simulink model "siude"  (Simulink 8.5)
settings: Solver=ode4  StartTime=0.0  StopTime=tstop  FixedStep=tstep  RelTol=1e-3
values from neighbouring files (symbols this model uses):
  bs_nom = Ka*Mn*dn*wa    (= -4.53426272631)    [dataude.m]
  kcm = 0.7    [dataude.m]
  kcn = 1.3    [dataude.m]
  rho = 10    [dataude.m]
settings Model: Creator=Dr SE Talole  LastModifiedBy=Vish
settings OptimizationCC: InitFltsAndDblsToZero=on
settings DebuggingCC: SaveWithParameterizedLinksMsg=none  SignalResolutionControl=TryResolveAllWithWarning  SolverPrmCheckMsg=warning  MultiTaskDSMMsg=warning  MultiTaskCondExecSysMsg=none  FcnCallInpInsideContextMsg=UseLocalSettings
settings GRTTargetCC: TargetFcnLib=ansi_tfl_tmw.mat

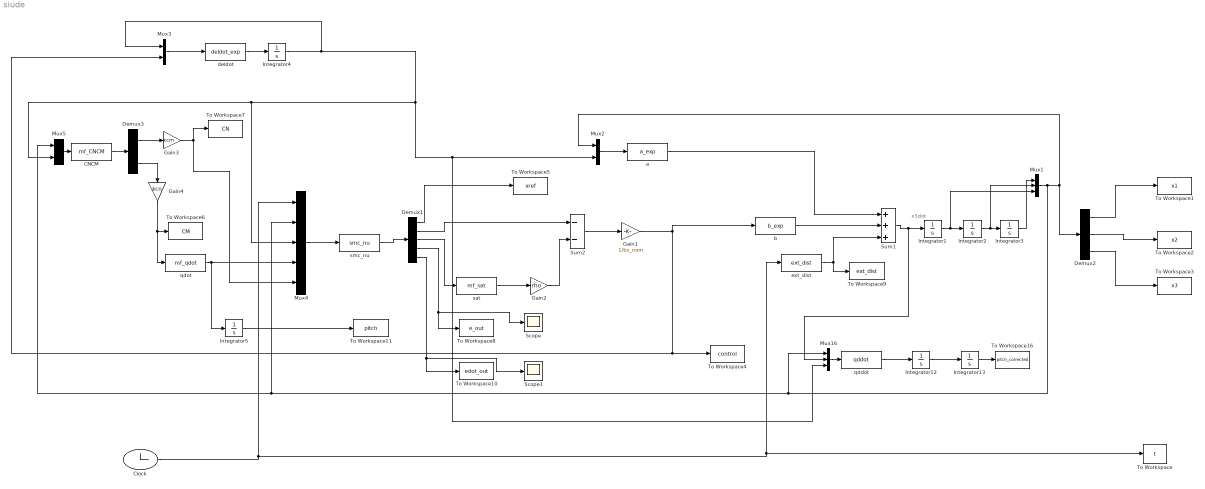
== system siude ==
  note: x3dot
  CNCM : MATLABFcn  MATLABFcn=mf_CNCM  OutputDimensions=2
  Clock : Clock
  Demux1 : Demux  Outputs=5
  Demux2 : Demux  Outputs=3
  Demux3 : Demux  Outputs=2
  Gain1 : Gain  Gain=1/bs_nom
  Gain2 : Gain  Gain=rho
  Gain3 : Gain  Gain=kcm
  Gain4 : Gain  Gain=kcn
  Integrator{1..5,12..13} (7 alike) : Integrator
  Mux1 : Mux  Inputs=3
  Mux16 : Mux  Inputs=3
  Mux2 : Mux  Inputs=2
  Mux3 : Mux  Inputs=2
  Mux4 : Mux  Inputs=5
  Mux5 : Mux  Inputs=2
  Scope : Scope
  Scope1 : Scope
  Sum1 : Sum  Inputs=+++
  Sum2 : Sum  Inputs=--
  To Workspace : ToWorkspace  VariableName=t  SampleTime=-1
  To Workspace1 : ToWorkspace  VariableName=x1  SampleTime=-1
  To Workspace10 : ToWorkspace  VariableName=edot_out  SampleTime=-1
  To Workspace11 : ToWorkspace  VariableName=pitch  SampleTime=-1
  To Workspace16 : ToWorkspace  VariableName=pitch_corrected  SampleTime=-1
  To Workspace2 : ToWorkspace  VariableName=x2  SampleTime=-1
  To Workspace3 : ToWorkspace  VariableName=x3  SampleTime=-1
  To Workspace4 : ToWorkspace  VariableName=control  SampleTime=-1
  To Workspace5 : ToWorkspace  VariableName=xref  SampleTime=-1
  To Workspace6 : ToWorkspace  VariableName=CM  SampleTime=-1
  To Workspace7 : ToWorkspace  VariableName=CN  SampleTime=-1
  To Workspace8 : ToWorkspace  VariableName=e_out  SampleTime=-1
  To Workspace9 : ToWorkspace  VariableName=ext_dist  SampleTime=-1
  a : MATLABFcn  MATLABFcn=a_exp  OutputDimensions=1
  b : MATLABFcn  MATLABFcn=b_exp  OutputDimensions=1
  deldot : MATLABFcn  MATLABFcn=deldot_exp  OutputDimensions=1
  "ext_dist " : MATLABFcn  MATLABFcn=ext_dist  OutputDimensions=1
  qddot : MATLABFcn  MATLABFcn=qddot  OutputDimensions=1
  qdot : MATLABFcn  MATLABFcn=mf_qdot  OutputDimensions=1
  sat : MATLABFcn  MATLABFcn=mf_sat  OutputDimensions=1
  smc_nu : MATLABFcn  MATLABFcn=smc_nu  OutputDimensions=5
  wires:
  Integrator3/1 -> Mux1/1
  Sum2/1 -> Gain1/1
  Demux1/1 -> To Workspace5/1
  Integrator2/1 -> Mux1/2, Integrator3/1
  Integrator1/1 -> Mux1/3, Integrator2/1
  Demux2/2 -> To Workspace2/1
  a/1 -> Sum1/1
  Mux2/1 -> a/1
  Mux3/1 -> deldot/1
  deldot/1 -> Integrator4/1
  Demux2/3 -> To Workspace3/1
  Gain1/1 -> b/1, To Workspace4/1, Mux3/2
  Demux2/1 -> To Workspace1/1
  b/1 -> Sum1/2
  "ext_dist "/1 -> Sum1/3, To Workspace9/1
  smc_nu/1 -> Demux1/1
  Demux1/2 -> Sum2/1
  Mux4/1 -> smc_nu/1
  Clock/1 -> Mux4/1, "ext_dist "/1, To Workspace/1
  qdot/1 -> Integrator5/1, Mux4/4
  Mux5/1 -> CNCM/1
  CNCM/1 -> Demux3/1
  Demux1/3 -> sat/1
  sat/1 -> Gain2/1
  Gain2/1 -> Sum2/2
  Demux3/2 -> Gain4/1
  Gain4/1 -> qdot/1, To Workspace6/1
  Demux3/1 -> Gain3/1
  Gain3/1 -> Mux4/5, To Workspace7/1
  Demux1/4 -> Scope/1, To Workspace8/1
  Demux1/5 -> To Workspace10/1, Scope1/1
  Integrator5/1 -> To Workspace11/1
  Integrator4/1 -> Mux4/3, Mux5/2, Mux16/3, Mux2/2, Mux3/1
  Sum1/1 -> Mux16/2, Integrator1/1
  Mux1/1 -> Mux16/1, Mux4/2, Mux5/1, Mux2/1, Demux2/1
  Mux16/1 -> qddot/1
  qddot/1 -> Integrator12/1
  Integrator12/1 -> Integrator13/1
  Integrator13/1 -> To Workspace16/1
